simulink model "Frec_Nat_c_mk_2"  (R2020a)
settings: Solver=ode4  StartTime=0.0  StopTime=10  FixedStep=0.001  RelTol=1e-3
values from neighbouring files (symbols this model uses):
  F = [200    300     400       500     600    700     800     900 1000 1100 1200]    [k.m]    (also in wn.m = P3*e*w^2)
  k1 = k*E*I/(a^3)    [wn.m]
  Mt1 = M+m    [wn.m]
undefined symbols (not defined in the file or in its folder): k2, Mt2
libraries: simulink x2
settings Model: Creator=karli  LastModifiedBy=karli

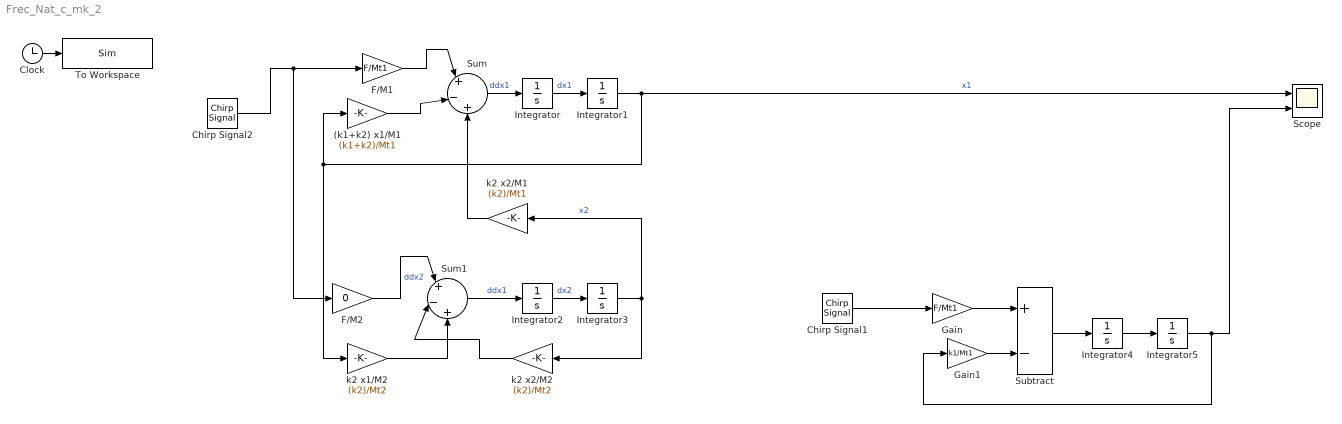
== system Frec_Nat_c_mk_2 ==
  (k1+k2) x1/M1 : Gain  Gain=(k1+k2)/Mt1
  Chirp Signal1 : simulink/Sources/Chirp Signal  f1=1  T=3  f2=40
  Chirp Signal2 : simulink/Sources/Chirp Signal  f1=1  T=3  f2=40
  Clock : Clock
  F/M1 : Gain  Gain=F/Mt1
  F/M2 : Gain  Gain=0
  Gain : Gain  Gain=F/Mt1
  Gain1 : Gain  Gain=k1/Mt1
  Integrator{,1..5} (6 alike) : Integrator
  Scope : Scope  NumInputPorts=2
  Subtract : Sum  Inputs=+-
  Sum : Sum  Inputs=|+|-|+
  Sum1 : Sum  Inputs=|+|-|+
  To Workspace : ToWorkspace  VariableName=Sim  SaveFormat=Structure  SampleTime=-1
  k2 x1/M2 : Gain  Gain=(k2)/Mt2
  k2 x2/M1 : Gain  Gain=(k2)/Mt1
  k2 x2/M2 : Gain  Gain=(k2)/Mt2
  wires:
  Clock/1 -> To Workspace/1
  Integrator/1 -> Integrator1/1  "dx1"
  Integrator1/1 -> k2 x1/M2/1, (k1+k2) x1/M1/1, Scope/1  "x1"
  F/M1/1 -> Sum/1
  Sum/1 -> Integrator/1  "ddx1"
  Integrator3/1 -> k2 x2/M2/1, k2 x2/M1/1  "x2"
  Integrator2/1 -> Integrator3/1  "dx2"
  k2 x2/M1/1 -> Sum/3
  (k1+k2) x1/M1/1 -> Sum/2
  Sum1/1 -> Integrator2/1  "ddx1"
  F/M2/1 -> Sum1/1  "ddx2"
  k2 x1/M2/1 -> Sum1/3
  k2 x2/M2/1 -> Sum1/2
  Subtract/1 -> Integrator4/1
  Integrator5/1 -> Gain1/1, Scope/2
  Gain/1 -> Subtract/1
  Gain1/1 -> Subtract/2
  Integrator4/1 -> Integrator5/1
  Chirp Signal2/1 -> F/M2/1, F/M1/1
  Chirp Signal1/1 -> Gain/1
